simulink model "rate_control"  (R2024a)
settings: Solver=FixedStepAuto  StartTime=0  StopTime=TimeStop  FixedStep=TimeStep  RelTol=1e-3
values from neighbouring files (symbols this model uses):
  D = Y_bar(:,1:m)    [Auxi_OKID_JXL.m]    (also in limit_cycle_est.m = 0:0.01:1)
  Desire_att = [0;0;90]    [run_pwpf.m]
  filter_gain_z = 2    [run_pwpf.m]
  filter_time_constant_x = 0.1    [run_pwpf.m]
  filter_time_constant_y = 0.1    [run_pwpf.m]
  filter_time_constant_z = 0.5    [run_pwpf.m]
  I = [0.619 -0.008 0;-0.008 0.782 0;0 0 1.226]    [limit_cycle_est.m]    (also in moment_calculation.m; run_pwpf.m = 1*[0.619 -0.008 0;-0.008 0.782 0;0 0 1.226])
  initial_condition = [20;20;0]    [run_pwpf.m]
  Schimitt_Lower_bound_x = 0.15    [run_pwpf.m]
  Schimitt_Lower_bound_y = 0.15    [run_pwpf.m]
  Schimitt_Lower_bound_z = 0.15    [run_pwpf.m]
  Schimitt_Upper_bound_x = 0.5    [run_pwpf.m]
  Schimitt_Upper_bound_y = 0.5    [run_pwpf.m]
  Schimitt_Upper_bound_z = 3    [run_pwpf.m]
  Thruster_mom_x = 0.35*0.5    (= 0.175)    [run_pwpf.m]
  Thruster_mom_y = 0.35*0.5    (= 0.175)    [run_pwpf.m]
  Thruster_mom_z = 0.35*0.5*2    (= 0.35)    [run_pwpf.m]
undefined symbols (not defined in the file or in its folder): aMode
libraries: slpidlib x6, simulink_extras x4, shared6dofsys x1, sharedutil x1
settings Model: Creator=cnsl  LastModifiedBy=s3928
settings DebuggingCC: AlgebraicLoopMsg=none
settings RTWCC: GPUComputeCapability=3.5

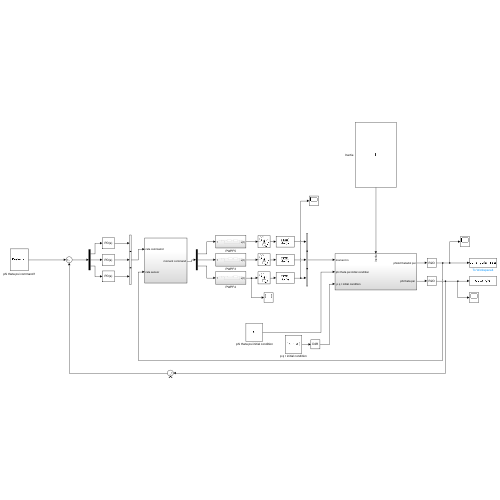
[thumbnail: Simulink's stored preview of the top-level diagram]
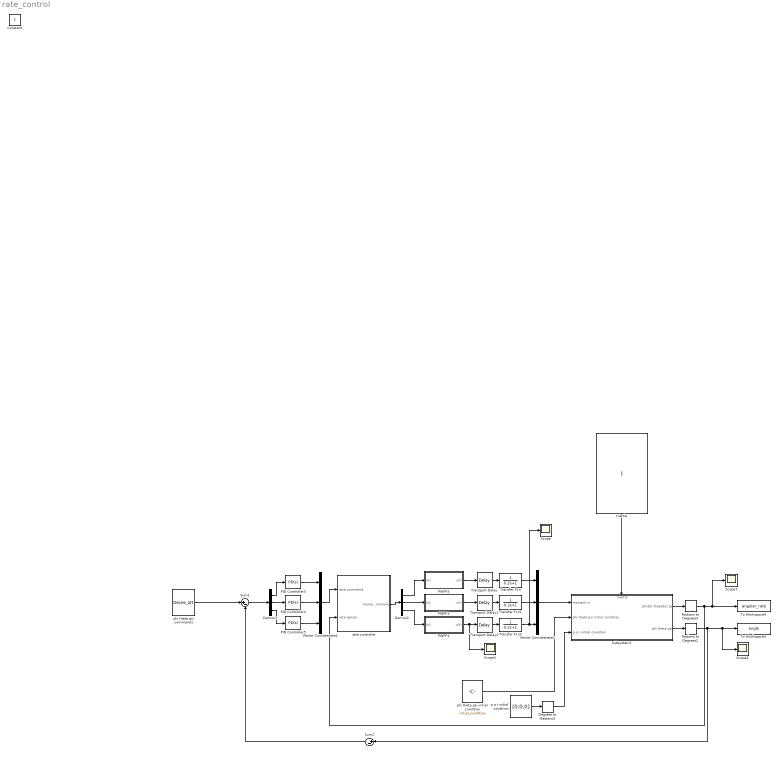
== system rate_control ==
  " phi theta psi initial condition" : Constant  Value=initial_condition
  Degrees to Radians3 : simulink_extras/Transformations/Degrees to Radians
  Demux1 : Demux  Outputs=3
  Demux2 : Demux  Outputs=3
  Inertie : Constant  Value=I
  PID Controller3 : slpidlib/PID Controller  Controller=PD  Form=Parallel  TimeDomain=Continuous-time  UseExternalTs=off  SampleTime=-1  IntegratorMethod=Forward Euler  FilterMethod=Forward Euler  ControllerParametersSource=internal  P=1  I=0.5  UseKiTs=off  D=2  UseExternalDerivativeSource=off  N=174.045132918495  UseFilter=on  TunerSelectOption=Transfer Function Based (PID Tuner App)  InitialConditionSource=internal  InitialConditionForIntegrator=0  InitialConditionForFilter=0  DifferentiatorICPrevScaledInput=0  ExternalReset=none  TrackingMode=off  Kt=1  LimitOutput=off  SatLimitsSource=internal  UpperSaturationLimit=inf  LowerSaturationLimit=-inf  LinearizeAsGain=on  AntiWindupMode=none  Kb=1  LimitIntegrator=off  UpperIntegratorSaturationLimit=inf  LowerIntegratorSaturationLimit=-inf  POutMin=[]  POutMax=[]  IOutMin=[]  IOutMax=[]  DOutMin=[]  DOutMax=[]  NOutMin=[]  NOutMax=[]  SumOutMin=[]  SumOutMax=[]  SaturationOutMin=[]  SaturationOutMax=[]  PParamMin=[]  PParamMax=[]  IParamMin=[]  IParamMax=[]  DParamMin=[]  DParamMax=[]  NParamMin=[]  NParamMax=[]  KbParamMin=[]  KbParamMax=[]  KtParamMin=[]  KtParamMax=[]  KbOutMin=[]  KbOutMax=[]  KtOutMin=[]  KtOutMax=[]  IntegratorOutMin=[]  IntegratorOutMax=[]  FilterOutMin=[]  FilterOutMax=[]  SumI1OutMin=[]  SumI1OutMax=[]  SumI2OutMin=[]  SumI2OutMax=[]  SumI3OutMin=[]  SumI3OutMax=[]  SumI4OutMin=[]  SumI4OutMax=[]  SumDOutMin=[]  SumDOutMax=[]  DifferentiatorOutMin=[]  DifferentiatorOutMax=[]  FilterDiffOutCoefMin=[]  FilterDiffOutCoefMax=[]  ReciprocalOutMin=[]  ReciprocalOutMax=[]  SumDenOutMin=[]  SumDenOutMax=[]  SumNumOutMin=[]  SumNumOutMax=[]  DivideOutMin=[]  DivideOutMax=[]  UdiffTsProdOutMin=[]  UdiffTsProdOutMax=[]  NTsProdOutMin=[]  NTsProdOutMax=[]  UintegralTsProdOutMin=[]  UintegralTsProdOutMax=[]  UngainTsProdOutMin=[]  UngainTsProdOutMax=[]  ClampingZeroOutDataTypeStr=Inherit: Inherit via back propagation  ClampingZeroOutMin=[]  ClampingZeroOutMax=[]  FilterDenConstantOutDataTypeStr=Inherit: Inherit via back propagation  FilterDenConstantOutMin=[]  FilterDenConstantOutMax=[]  PCopyOutDataTypeStr=Inherit: Inherit via back propagation  PCopyOutMin=[]  PCopyOutMax=[]  NCopyOutDataTypeStr=Inherit: Inherit via back propagation  NCopyOutMin=[]  NCopyOutMax=[]  IntegratorContinuousStateAttributes=''  IntegratorStateMustResolveToSignalObject=off  IntegratorRTWStateStorageClass=Auto  FilterContinuousStateAttributes=''  FilterStateMustResolveToSignalObject=off  FilterRTWStateStorageClass=Auto  ParallelPVariant=InternalParameters  IdealPVariant=Disabled  IVariant=Disabled  DVariant=InternalParameters  IntegratorVariant=Disabled  SatVariant=Disabled  AWVariant=Disabled  PCopyVariant=Disabled  TRVariant=Disabled  FdbkBlocksVariant=Forward  IdealPFdbkVariant=Disabled  SatFdbkVariant=Disabled  DerivativeFilterVariant=ContFilter  NVariant=InternalParameters  NCopyVariant=Disabled  FilterICVariant=InternalICsFilter  IntegratorICVariant=Disabled  ExternalResetVariant=Disabled  TRSumVariant=Passthrough  SumFdbkVariant=Disabled  SumVariant=Sum_PD  TsampFilterVariant=InternalTs  TsampNgainVariant=Passthrough  TsampIntegralVariant=Disabled_SignalSpec  ExternalSaturationOutDataTypeStr=Inherit: Same as second input  DerivativeSourceVariant=ErrorSignal
  PID Controller4 : slpidlib/PID Controller  Controller=PD  Form=Parallel  TimeDomain=Continuous-time  UseExternalTs=off  SampleTime=-1  IntegratorMethod=Forward Euler  FilterMethod=Forward Euler  ControllerParametersSource=internal  P=1  I=0.1  UseKiTs=off  D=2  UseExternalDerivativeSource=off  N=1000  UseFilter=on  TunerSelectOption=Transfer Function Based (PID Tuner App)  InitialConditionSource=internal  InitialConditionForIntegrator=0  InitialConditionForFilter=0  DifferentiatorICPrevScaledInput=0  ExternalReset=none  TrackingMode=off  Kt=1  LimitOutput=off  SatLimitsSource=internal  UpperSaturationLimit=inf  LowerSaturationLimit=-inf  LinearizeAsGain=on  AntiWindupMode=none  Kb=1  LimitIntegrator=off  UpperIntegratorSaturationLimit=inf  LowerIntegratorSaturationLimit=-inf  POutMin=[]  POutMax=[]  IOutMin=[]  IOutMax=[]  DOutMin=[]  DOutMax=[]  NOutMin=[]  NOutMax=[]  SumOutMin=[]  SumOutMax=[]  SaturationOutMin=[]  SaturationOutMax=[]  PParamMin=[]  PParamMax=[]  IParamMin=[]  IParamMax=[]  DParamMin=[]  DParamMax=[]  NParamMin=[]  NParamMax=[]  KbParamMin=[]  KbParamMax=[]  KtParamMin=[]  KtParamMax=[]  KbOutMin=[]  KbOutMax=[]  KtOutMin=[]  KtOutMax=[]  IntegratorOutMin=[]  IntegratorOutMax=[]  FilterOutMin=[]  FilterOutMax=[]  SumI1OutMin=[]  SumI1OutMax=[]  SumI2OutMin=[]  SumI2OutMax=[]  SumI3OutMin=[]  SumI3OutMax=[]  SumI4OutMin=[]  SumI4OutMax=[]  SumDOutMin=[]  SumDOutMax=[]  DifferentiatorOutMin=[]  DifferentiatorOutMax=[]  FilterDiffOutCoefMin=[]  FilterDiffOutCoefMax=[]  ReciprocalOutMin=[]  ReciprocalOutMax=[]  SumDenOutMin=[]  SumDenOutMax=[]  SumNumOutMin=[]  SumNumOutMax=[]  DivideOutMin=[]  DivideOutMax=[]  UdiffTsProdOutMin=[]  UdiffTsProdOutMax=[]  NTsProdOutMin=[]  NTsProdOutMax=[]  UintegralTsProdOutMin=[]  UintegralTsProdOutMax=[]  UngainTsProdOutMin=[]  UngainTsProdOutMax=[]  ClampingZeroOutDataTypeStr=Inherit: Inherit via back propagation  ClampingZeroOutMin=[]  ClampingZeroOutMax=[]  FilterDenConstantOutDataTypeStr=Inherit: Inherit via back propagation  FilterDenConstantOutMin=[]  FilterDenConstantOutMax=[]  PCopyOutDataTypeStr=Inherit: Inherit via back propagation  PCopyOutMin=[]  PCopyOutMax=[]  NCopyOutDataTypeStr=Inherit: Inherit via back propagation  NCopyOutMin=[]  NCopyOutMax=[]  IntegratorContinuousStateAttributes=''  IntegratorStateMustResolveToSignalObject=off  IntegratorRTWStateStorageClass=Auto  FilterContinuousStateAttributes=''  FilterStateMustResolveToSignalObject=off  FilterRTWStateStorageClass=Auto  ParallelPVariant=InternalParameters  IdealPVariant=Disabled  IVariant=Disabled  DVariant=InternalParameters  IntegratorVariant=Disabled  SatVariant=Disabled  AWVariant=Disabled  PCopyVariant=Disabled  TRVariant=Disabled  FdbkBlocksVariant=Forward  IdealPFdbkVariant=Disabled  SatFdbkVariant=Disabled  DerivativeFilterVariant=ContFilter  NVariant=InternalParameters  NCopyVariant=Disabled  FilterICVariant=InternalICsFilter  IntegratorICVariant=Disabled  ExternalResetVariant=Disabled  TRSumVariant=Passthrough  SumFdbkVariant=Disabled  SumVariant=Sum_PD  TsampFilterVariant=InternalTs  TsampNgainVariant=Passthrough  TsampIntegralVariant=Disabled_SignalSpec  ExternalSaturationOutDataTypeStr=Inherit: Same as second input  DerivativeSourceVariant=ErrorSignal
  PID Controller5 : slpidlib/PID Controller  Controller=PD  Form=Parallel  TimeDomain=Continuous-time  UseExternalTs=off  SampleTime=-1  IntegratorMethod=Forward Euler  FilterMethod=Forward Euler  ControllerParametersSource=internal  P=1  I=0.2  UseKiTs=off  D=2  UseExternalDerivativeSource=off  N=1142.8279760416  UseFilter=on  TunerSelectOption=Transfer Function Based (PID Tuner App)  InitialConditionSource=internal  InitialConditionForIntegrator=0  InitialConditionForFilter=0  DifferentiatorICPrevScaledInput=0  ExternalReset=none  TrackingMode=off  Kt=1  LimitOutput=off  SatLimitsSource=internal  UpperSaturationLimit=inf  LowerSaturationLimit=-inf  LinearizeAsGain=on  AntiWindupMode=none  Kb=1  LimitIntegrator=off  UpperIntegratorSaturationLimit=inf  LowerIntegratorSaturationLimit=-inf  POutMin=[]  POutMax=[]  IOutMin=[]  IOutMax=[]  DOutMin=[]  DOutMax=[]  NOutMin=[]  NOutMax=[]  SumOutMin=[]  SumOutMax=[]  SaturationOutMin=[]  SaturationOutMax=[]  PParamMin=[]  PParamMax=[]  IParamMin=[]  IParamMax=[]  DParamMin=[]  DParamMax=[]  NParamMin=[]  NParamMax=[]  KbParamMin=[]  KbParamMax=[]  KtParamMin=[]  KtParamMax=[]  KbOutMin=[]  KbOutMax=[]  KtOutMin=[]  KtOutMax=[]  IntegratorOutMin=[]  IntegratorOutMax=[]  FilterOutMin=[]  FilterOutMax=[]  SumI1OutMin=[]  SumI1OutMax=[]  SumI2OutMin=[]  SumI2OutMax=[]  SumI3OutMin=[]  SumI3OutMax=[]  SumI4OutMin=[]  SumI4OutMax=[]  SumDOutMin=[]  SumDOutMax=[]  DifferentiatorOutMin=[]  DifferentiatorOutMax=[]  FilterDiffOutCoefMin=[]  FilterDiffOutCoefMax=[]  ReciprocalOutMin=[]  ReciprocalOutMax=[]  SumDenOutMin=[]  SumDenOutMax=[]  SumNumOutMin=[]  SumNumOutMax=[]  DivideOutMin=[]  DivideOutMax=[]  UdiffTsProdOutMin=[]  UdiffTsProdOutMax=[]  NTsProdOutMin=[]  NTsProdOutMax=[]  UintegralTsProdOutMin=[]  UintegralTsProdOutMax=[]  UngainTsProdOutMin=[]  UngainTsProdOutMax=[]  ClampingZeroOutDataTypeStr=Inherit: Inherit via back propagation  ClampingZeroOutMin=[]  ClampingZeroOutMax=[]  FilterDenConstantOutDataTypeStr=Inherit: Inherit via back propagation  FilterDenConstantOutMin=[]  FilterDenConstantOutMax=[]  PCopyOutDataTypeStr=Inherit: Inherit via back propagation  PCopyOutMin=[]  PCopyOutMax=[]  NCopyOutDataTypeStr=Inherit: Inherit via back propagation  NCopyOutMin=[]  NCopyOutMax=[]  IntegratorContinuousStateAttributes=''  IntegratorStateMustResolveToSignalObject=off  IntegratorRTWStateStorageClass=Auto  FilterContinuousStateAttributes=''  FilterStateMustResolveToSignalObject=off  FilterRTWStateStorageClass=Auto  ParallelPVariant=InternalParameters  IdealPVariant=Disabled  IVariant=Disabled  DVariant=InternalParameters  IntegratorVariant=Disabled  SatVariant=Disabled  AWVariant=Disabled  PCopyVariant=Disabled  TRVariant=Disabled  FdbkBlocksVariant=Forward  IdealPFdbkVariant=Disabled  SatFdbkVariant=Disabled  DerivativeFilterVariant=ContFilter  NVariant=InternalParameters  NCopyVariant=Disabled  FilterICVariant=InternalICsFilter  IntegratorICVariant=Disabled  ExternalResetVariant=Disabled  TRSumVariant=Passthrough  SumFdbkVariant=Disabled  SumVariant=Sum_PD  TsampFilterVariant=InternalTs  TsampNgainVariant=Passthrough  TsampIntegralVariant=Disabled_SignalSpec  ExternalSaturationOutDataTypeStr=Inherit: Same as second input  DerivativeSourceVariant=ErrorSignal
  PWPF3 : Subsystem
  PWPF4 : Subsystem
  PWPF5 : Subsystem
  Radians to Degrees2 : simulink_extras/Transformations/Radians to Degrees
  Radians to Degrees3 : simulink_extras/Transformations/Radians to Degrees
  Scope{,1,3,7} (4 alike) : Scope
  Subsystem1 : Subsystem
      settings: PortSchema="{\"entries\":[{\"content\":{\"sides\":[{\"content\":{\"connectorIds\":[\"In1\",\"In2\",\"In3\"]},\"type\":\"ConnectorPlacement.EquallySpacedRectSide\",\"uuid\":\"69618b35-6270-4939-99e0-c93e8a624a88\"},{\"content\":{\"connectorIds\":[\"Out1\",\"Out2\"],\"side\":\"RIGHT\"},\"type\":\"ConnectorPlacement.EquallySpacedRectSide\",\"uuid\":\"dd38394a-61d4-4afa-a4aa-1d349921c55b\"},{\"content\":{\"connectorIds\":[\"In4\"],\"side\":\"TOP\"},\"type\":\"ConnectorPlacement.EquallySpacedRectSide\",\"uuid\":\"df8b2583-6705-491e-930f-9a3acb03c8ce\"}]},\"type\":\"ConnectorPlacement.EquallySpacedConnector\",\"uuid\":\"e8247de4-3909-4e19-8e9e-570170f34f7b\"}],\"packageUris\":[\"http://schema.mathworks.com/mf0/Connector/R2020b\"],\"version\":\"1.0\"}"
  Sum1 : Sum  Inputs=|+-
  Sum2 : Sum  Inputs=|+-
  To Workspace3 : ToWorkspace  VariableName=angle  SaveFormat=Timeseries  SampleTime=-1
  To Workspace4 : ToWorkspace  VariableName=angular_rate  SaveFormat=Timeseries  SampleTime=-1
  Transfer Fcn : TransferFcn  Denominator=[0.2 1]
  Transfer Fcn1 : TransferFcn  Denominator=[0.2 1]
  Transfer Fcn2 : TransferFcn  Denominator=[0.2 1]
  Transport Delay : TransportDelay  DelayTime=0.05
  Transport Delay1 : TransportDelay  DelayTime=0.05
  Transport Delay2 : TransportDelay  DelayTime=0.05
  Vector Concatenate1 : Concatenate  NumInputs=3
  Vector Concatenate2 : Concatenate  NumInputs=3
  p q r initial condition : Constant  Value=[0;0;0]
  phi theta psi command1 : Constant  Value=Desire_att
  rate controller : Subsystem
  Constant : Constant  IOType=siggen
  wires:
  Sum1/1 -> Demux1/1
  Demux1/2 -> PID Controller4/1
  Demux1/3 -> PID Controller5/1
  Subsystem1/1(phidot thetadot psi) -> Radians to Degrees3/1
  Demux1/1 -> PID Controller3/1
  phi theta psi command1/1 -> Sum1/1
  Subsystem1/2("phi theta psi ") -> Radians to Degrees2/1
  p q r initial condition/1 -> Degrees to Radians3/1
  Inertie/1 -> Subsystem1/4(inertia)
  Radians to Degrees3/1 -> rate controller/2(rate sensor), Scope7/1, To Workspace4/1
  " phi theta psi initial condition"/1 -> Subsystem1/2("phi theta psi initial condition ")
  Degrees to Radians3/1 -> Subsystem1/3(" p q r initial condition")
  Radians to Degrees2/1 -> Scope3/1, To Workspace3/1, Sum2/1
  PID Controller3/1 -> Vector Concatenate1/1
  PID Controller4/1 -> Vector Concatenate1/2
  PID Controller5/1 -> Vector Concatenate1/3
  Vector Concatenate1/1 -> rate controller/1(rate commamd)
  Demux2/1 -> PWPF5/1(In1)
  Demux2/3 -> PWPF4/1(In1)
  Demux2/2 -> PWPF3/1(In1)
  rate controller/1(moment command) -> Demux2/1
  Sum2/1 -> Sum1/2
  Vector Concatenate2/1 -> Subsystem1/1(moment in)
  Transport Delay/1 -> Transfer Fcn/1
  Transfer Fcn/1 -> Vector Concatenate2/1
  PWPF5/1(u(t)) -> Transport Delay/1
  Transport Delay1/1 -> Transfer Fcn1/1
  Transport Delay2/1 -> Transfer Fcn2/1
  Transfer Fcn1/1 -> Vector Concatenate2/2
  Transfer Fcn2/1 -> Scope/1, Vector Concatenate2/3
  PWPF3/1(u(t)) -> Transport Delay1/1
  PWPF4/1(u(t)) -> Scope1/1, Transport Delay2/1

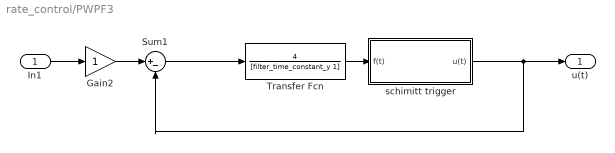
== system rate_control/PWPF3 ==
  In1 : Inport
  Gain2 : Gain
  Sum1 : Sum  Inputs=|+-
  Transfer Fcn : TransferFcn  Numerator=[4]  Denominator=[filter_time_constant_y 1]
  schimitt trigger : Subsystem
  u(t) : Outport
  wires:
  In1/1 -> Gain2/1
  Gain2/1 -> Sum1/1
  schimitt trigger/1(u(t)) -> u(t)/1, Sum1/2
  Sum1/1 -> Transfer Fcn/1
  Transfer Fcn/1 -> schimitt trigger/1(f(t))

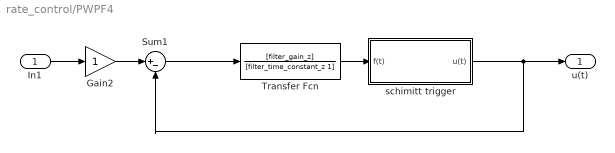
== system rate_control/PWPF4 ==
  In1 : Inport
  Gain2 : Gain
  Sum1 : Sum  Inputs=|+-
  Transfer Fcn : TransferFcn  Numerator=[filter_gain_z]  Denominator=[filter_time_constant_z 1]
  schimitt trigger : Subsystem
  u(t) : Outport
  wires:
  Transfer Fcn/1 -> schimitt trigger/1(f(t))
  Sum1/1 -> Transfer Fcn/1
  schimitt trigger/1(u(t)) -> Sum1/2, u(t)/1
  Gain2/1 -> Sum1/1
  In1/1 -> Gain2/1

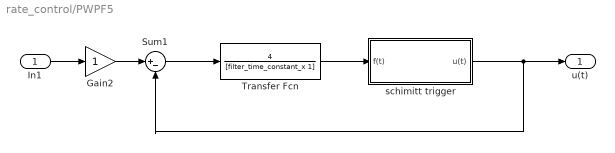
== system rate_control/PWPF5 ==
  In1 : Inport
  Gain2 : Gain
  Sum1 : Sum  Inputs=|+-
  Transfer Fcn : TransferFcn  Numerator=[4]  Denominator=[filter_time_constant_x 1]
  schimitt trigger : Subsystem
  u(t) : Outport
  wires:
  Transfer Fcn/1 -> schimitt trigger/1(f(t))
  Sum1/1 -> Transfer Fcn/1
  schimitt trigger/1(u(t)) -> Sum1/2, u(t)/1
  Gain2/1 -> Sum1/1
  In1/1 -> Gain2/1

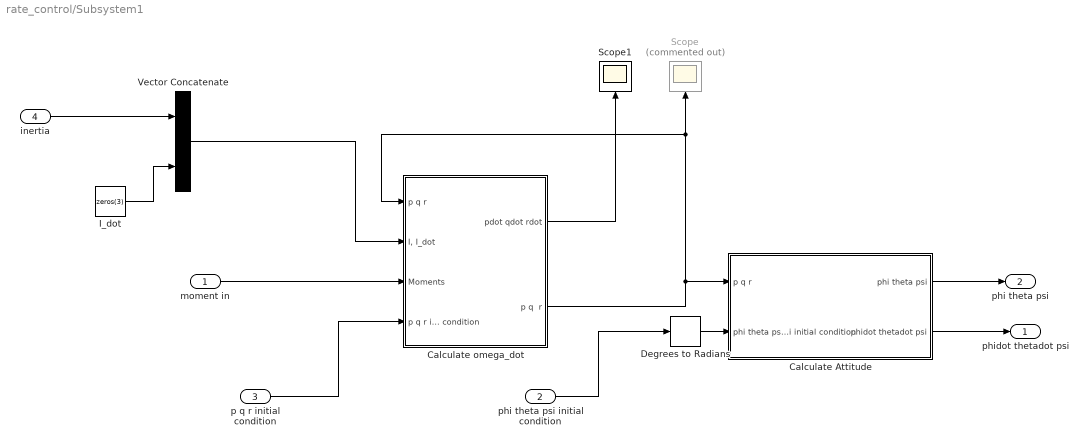
== system rate_control/Subsystem1 ==
  moment in : Inport
  "phi theta psi initial condition " : Inport  Port=2
  " p q r initial condition" : Inport  Port=3
  inertia : Inport  Port=4
  "Calculate Attitude " : Subsystem
  Calculate omega_dot : Subsystem  AncestorBlock=shared6dofsys/Calculate omega_dot  mask{aMode=aMode}
      mask init:
      | if aerosharedtest(gcb)
      |     aerosharedicon('shared');
      | else
      |     sharedautoicon('shared');
      | end
      settings: LibrarySourceBlock=shared6dofsys/Calculate omega_dot
  Degrees to Radians : simulink_extras/Transformations/Degrees to Radians
  I_dot : Constant  Value=zeros(3)
  Scope : Scope  Commented=on
  Scope1 : Scope
  Vector Concatenate : Concatenate  Mode=Multidimensional array
  phidot thetadot psi : Outport
  "phi theta psi " : Outport  Port=2
  wires:
  Vector Concatenate/1 -> Calculate omega_dot/2("I, I_dot")
  inertia/1 -> Vector Concatenate/1
  Calculate omega_dot/2(p q  r) -> Scope/1, Calculate omega_dot/1(p q r), "Calculate Attitude "/1(p q r)
  I_dot/1 -> Vector Concatenate/2
  " p q r initial condition"/1 -> Calculate omega_dot/4(p q r initial condition)
  "Calculate Attitude "/1("phi theta psi ") -> "phi theta psi "/1
  Degrees to Radians/1 -> "Calculate Attitude "/2("phi theta psi initial condition ")
  "phi theta psi initial condition "/1 -> Degrees to Radians/1
  "Calculate Attitude "/2(phidot thetadot psi) -> phidot thetadot psi/1
  Calculate omega_dot/1(pdot qdot rdot) -> Scope1/1
  moment in/1 -> Calculate omega_dot/3(Moments)

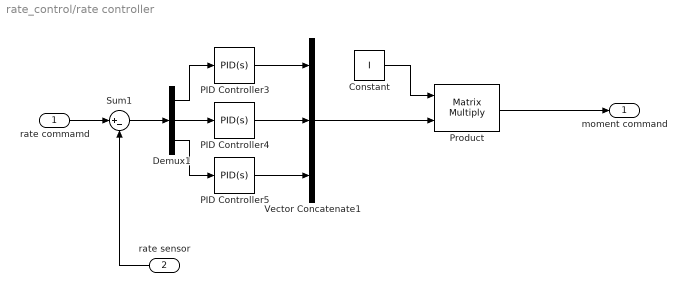
== system rate_control/rate controller ==
  rate commamd : Inport
  rate sensor : Inport  Port=2
  Constant : Constant  Value=I
  Demux1 : Demux  Outputs=3
  PID Controller3 : slpidlib/PID Controller  Controller=PID  Form=Parallel  TimeDomain=Continuous-time  UseExternalTs=off  SampleTime=-1  IntegratorMethod=Forward Euler  FilterMethod=Forward Euler  ControllerParametersSource=internal  P=2  I=0.25  UseKiTs=off  D=1  UseExternalDerivativeSource=off  N=100  UseFilter=on  TunerSelectOption=Transfer Function Based (PID Tuner App)  InitialConditionSource=internal  InitialConditionForIntegrator=0  InitialConditionForFilter=0  DifferentiatorICPrevScaledInput=0  ExternalReset=none  TrackingMode=off  Kt=1  LimitOutput=off  SatLimitsSource=internal  UpperSaturationLimit=inf  LowerSaturationLimit=-inf  LinearizeAsGain=on  AntiWindupMode=none  Kb=1  LimitIntegrator=off  UpperIntegratorSaturationLimit=inf  LowerIntegratorSaturationLimit=-inf  POutMin=[]  POutMax=[]  IOutMin=[]  IOutMax=[]  DOutMin=[]  DOutMax=[]  NOutMin=[]  NOutMax=[]  SumOutMin=[]  SumOutMax=[]  SaturationOutMin=[]  SaturationOutMax=[]  PParamMin=[]  PParamMax=[]  IParamMin=[]  IParamMax=[]  DParamMin=[]  DParamMax=[]  NParamMin=[]  NParamMax=[]  KbParamMin=[]  KbParamMax=[]  KtParamMin=[]  KtParamMax=[]  KbOutMin=[]  KbOutMax=[]  KtOutMin=[]  KtOutMax=[]  IntegratorOutMin=[]  IntegratorOutMax=[]  FilterOutMin=[]  FilterOutMax=[]  SumI1OutMin=[]  SumI1OutMax=[]  SumI2OutMin=[]  SumI2OutMax=[]  SumI3OutMin=[]  SumI3OutMax=[]  SumI4OutMin=[]  SumI4OutMax=[]  SumDOutMin=[]  SumDOutMax=[]  DifferentiatorOutMin=[]  DifferentiatorOutMax=[]  FilterDiffOutCoefMin=[]  FilterDiffOutCoefMax=[]  ReciprocalOutMin=[]  ReciprocalOutMax=[]  SumDenOutMin=[]  SumDenOutMax=[]  SumNumOutMin=[]  SumNumOutMax=[]  DivideOutMin=[]  DivideOutMax=[]  UdiffTsProdOutMin=[]  UdiffTsProdOutMax=[]  NTsProdOutMin=[]  NTsProdOutMax=[]  UintegralTsProdOutMin=[]  UintegralTsProdOutMax=[]  UngainTsProdOutMin=[]  UngainTsProdOutMax=[]  ClampingZeroOutDataTypeStr=Inherit: Inherit via back propagation  ClampingZeroOutMin=[]  ClampingZeroOutMax=[]  FilterDenConstantOutDataTypeStr=Inherit: Inherit via back propagation  FilterDenConstantOutMin=[]  FilterDenConstantOutMax=[]  PCopyOutDataTypeStr=Inherit: Inherit via back propagation  PCopyOutMin=[]  PCopyOutMax=[]  NCopyOutDataTypeStr=Inherit: Inherit via back propagation  NCopyOutMin=[]  NCopyOutMax=[]  IntegratorContinuousStateAttributes=''  IntegratorStateMustResolveToSignalObject=off  IntegratorRTWStateStorageClass=Auto  FilterContinuousStateAttributes=''  FilterStateMustResolveToSignalObject=off  FilterRTWStateStorageClass=Auto  ParallelPVariant=InternalParameters  IdealPVariant=Disabled  IVariant=InternalParameters  DVariant=InternalParameters  IntegratorVariant=Continuous  SatVariant=Disabled  AWVariant=Passthrough  PCopyVariant=Disabled  TRVariant=Disabled  FdbkBlocksVariant=Forward  IdealPFdbkVariant=Disabled  SatFdbkVariant=Disabled  DerivativeFilterVariant=ContFilter  NVariant=InternalParameters  NCopyVariant=Disabled  FilterICVariant=InternalICsFilter  IntegratorICVariant=InternalICs  ExternalResetVariant=Disabled  TRSumVariant=Passthrough  SumFdbkVariant=Disabled  SumVariant=Sum_PID  TsampFilterVariant=InternalTs  TsampNgainVariant=Passthrough  TsampIntegralVariant=Disabled_SignalSpec  ExternalSaturationOutDataTypeStr=Inherit: Same as second input  DerivativeSourceVariant=ErrorSignal
  PID Controller4 : slpidlib/PID Controller  Controller=PID  Form=Parallel  TimeDomain=Continuous-time  UseExternalTs=off  SampleTime=-1  IntegratorMethod=Forward Euler  FilterMethod=Forward Euler  ControllerParametersSource=internal  P=2  I=0.25  UseKiTs=off  D=1  UseExternalDerivativeSource=off  N=100  UseFilter=on  TunerSelectOption=Transfer Function Based (PID Tuner App)  InitialConditionSource=internal  InitialConditionForIntegrator=0  InitialConditionForFilter=0  DifferentiatorICPrevScaledInput=0  ExternalReset=none  TrackingMode=off  Kt=1  LimitOutput=off  SatLimitsSource=internal  UpperSaturationLimit=inf  LowerSaturationLimit=-inf  LinearizeAsGain=on  AntiWindupMode=none  Kb=1  LimitIntegrator=off  UpperIntegratorSaturationLimit=inf  LowerIntegratorSaturationLimit=-inf  POutMin=[]  POutMax=[]  IOutMin=[]  IOutMax=[]  DOutMin=[]  DOutMax=[]  NOutMin=[]  NOutMax=[]  SumOutMin=[]  SumOutMax=[]  SaturationOutMin=[]  SaturationOutMax=[]  PParamMin=[]  PParamMax=[]  IParamMin=[]  IParamMax=[]  DParamMin=[]  DParamMax=[]  NParamMin=[]  NParamMax=[]  KbParamMin=[]  KbParamMax=[]  KtParamMin=[]  KtParamMax=[]  KbOutMin=[]  KbOutMax=[]  KtOutMin=[]  KtOutMax=[]  IntegratorOutMin=[]  IntegratorOutMax=[]  FilterOutMin=[]  FilterOutMax=[]  SumI1OutMin=[]  SumI1OutMax=[]  SumI2OutMin=[]  SumI2OutMax=[]  SumI3OutMin=[]  SumI3OutMax=[]  SumI4OutMin=[]  SumI4OutMax=[]  SumDOutMin=[]  SumDOutMax=[]  DifferentiatorOutMin=[]  DifferentiatorOutMax=[]  FilterDiffOutCoefMin=[]  FilterDiffOutCoefMax=[]  ReciprocalOutMin=[]  ReciprocalOutMax=[]  SumDenOutMin=[]  SumDenOutMax=[]  SumNumOutMin=[]  SumNumOutMax=[]  DivideOutMin=[]  DivideOutMax=[]  UdiffTsProdOutMin=[]  UdiffTsProdOutMax=[]  NTsProdOutMin=[]  NTsProdOutMax=[]  UintegralTsProdOutMin=[]  UintegralTsProdOutMax=[]  UngainTsProdOutMin=[]  UngainTsProdOutMax=[]  ClampingZeroOutDataTypeStr=Inherit: Inherit via back propagation  ClampingZeroOutMin=[]  ClampingZeroOutMax=[]  FilterDenConstantOutDataTypeStr=Inherit: Inherit via back propagation  FilterDenConstantOutMin=[]  FilterDenConstantOutMax=[]  PCopyOutDataTypeStr=Inherit: Inherit via back propagation  PCopyOutMin=[]  PCopyOutMax=[]  NCopyOutDataTypeStr=Inherit: Inherit via back propagation  NCopyOutMin=[]  NCopyOutMax=[]  IntegratorContinuousStateAttributes=''  IntegratorStateMustResolveToSignalObject=off  IntegratorRTWStateStorageClass=Auto  FilterContinuousStateAttributes=''  FilterStateMustResolveToSignalObject=off  FilterRTWStateStorageClass=Auto  ParallelPVariant=InternalParameters  IdealPVariant=Disabled  IVariant=InternalParameters  DVariant=InternalParameters  IntegratorVariant=Continuous  SatVariant=Disabled  AWVariant=Passthrough  PCopyVariant=Disabled  TRVariant=Disabled  FdbkBlocksVariant=Forward  IdealPFdbkVariant=Disabled  SatFdbkVariant=Disabled  DerivativeFilterVariant=ContFilter  NVariant=InternalParameters  NCopyVariant=Disabled  FilterICVariant=InternalICsFilter  IntegratorICVariant=InternalICs  ExternalResetVariant=Disabled  TRSumVariant=Passthrough  SumFdbkVariant=Disabled  SumVariant=Sum_PID  TsampFilterVariant=InternalTs  TsampNgainVariant=Passthrough  TsampIntegralVariant=Disabled_SignalSpec  ExternalSaturationOutDataTypeStr=Inherit: Same as second input  DerivativeSourceVariant=ErrorSignal
  PID Controller5 : slpidlib/PID Controller  Controller=PID  Form=Parallel  TimeDomain=Continuous-time  UseExternalTs=off  SampleTime=-1  IntegratorMethod=Forward Euler  FilterMethod=Forward Euler  ControllerParametersSource=internal  P=2  I=0.25  UseKiTs=off  D=1  UseExternalDerivativeSource=off  N=100  UseFilter=on  TunerSelectOption=Transfer Function Based (PID Tuner App)  InitialConditionSource=internal  InitialConditionForIntegrator=0  InitialConditionForFilter=0  DifferentiatorICPrevScaledInput=0  ExternalReset=none  TrackingMode=off  Kt=1  LimitOutput=off  SatLimitsSource=internal  UpperSaturationLimit=inf  LowerSaturationLimit=-inf  LinearizeAsGain=on  AntiWindupMode=none  Kb=1  LimitIntegrator=off  UpperIntegratorSaturationLimit=inf  LowerIntegratorSaturationLimit=-inf  POutMin=[]  POutMax=[]  IOutMin=[]  IOutMax=[]  DOutMin=[]  DOutMax=[]  NOutMin=[]  NOutMax=[]  SumOutMin=[]  SumOutMax=[]  SaturationOutMin=[]  SaturationOutMax=[]  PParamMin=[]  PParamMax=[]  IParamMin=[]  IParamMax=[]  DParamMin=[]  DParamMax=[]  NParamMin=[]  NParamMax=[]  KbParamMin=[]  KbParamMax=[]  KtParamMin=[]  KtParamMax=[]  KbOutMin=[]  KbOutMax=[]  KtOutMin=[]  KtOutMax=[]  IntegratorOutMin=[]  IntegratorOutMax=[]  FilterOutMin=[]  FilterOutMax=[]  SumI1OutMin=[]  SumI1OutMax=[]  SumI2OutMin=[]  SumI2OutMax=[]  SumI3OutMin=[]  SumI3OutMax=[]  SumI4OutMin=[]  SumI4OutMax=[]  SumDOutMin=[]  SumDOutMax=[]  DifferentiatorOutMin=[]  DifferentiatorOutMax=[]  FilterDiffOutCoefMin=[]  FilterDiffOutCoefMax=[]  ReciprocalOutMin=[]  ReciprocalOutMax=[]  SumDenOutMin=[]  SumDenOutMax=[]  SumNumOutMin=[]  SumNumOutMax=[]  DivideOutMin=[]  DivideOutMax=[]  UdiffTsProdOutMin=[]  UdiffTsProdOutMax=[]  NTsProdOutMin=[]  NTsProdOutMax=[]  UintegralTsProdOutMin=[]  UintegralTsProdOutMax=[]  UngainTsProdOutMin=[]  UngainTsProdOutMax=[]  ClampingZeroOutDataTypeStr=Inherit: Inherit via back propagation  ClampingZeroOutMin=[]  ClampingZeroOutMax=[]  FilterDenConstantOutDataTypeStr=Inherit: Inherit via back propagation  FilterDenConstantOutMin=[]  FilterDenConstantOutMax=[]  PCopyOutDataTypeStr=Inherit: Inherit via back propagation  PCopyOutMin=[]  PCopyOutMax=[]  NCopyOutDataTypeStr=Inherit: Inherit via back propagation  NCopyOutMin=[]  NCopyOutMax=[]  IntegratorContinuousStateAttributes=''  IntegratorStateMustResolveToSignalObject=off  IntegratorRTWStateStorageClass=Auto  FilterContinuousStateAttributes=''  FilterStateMustResolveToSignalObject=off  FilterRTWStateStorageClass=Auto  ParallelPVariant=InternalParameters  IdealPVariant=Disabled  IVariant=InternalParameters  DVariant=InternalParameters  IntegratorVariant=Continuous  SatVariant=Disabled  AWVariant=Passthrough  PCopyVariant=Disabled  TRVariant=Disabled  FdbkBlocksVariant=Forward  IdealPFdbkVariant=Disabled  SatFdbkVariant=Disabled  DerivativeFilterVariant=ContFilter  NVariant=InternalParameters  NCopyVariant=Disabled  FilterICVariant=InternalICsFilter  IntegratorICVariant=InternalICs  ExternalResetVariant=Disabled  TRSumVariant=Passthrough  SumFdbkVariant=Disabled  SumVariant=Sum_PID  TsampFilterVariant=InternalTs  TsampNgainVariant=Passthrough  TsampIntegralVariant=Disabled_SignalSpec  ExternalSaturationOutDataTypeStr=Inherit: Same as second input  DerivativeSourceVariant=ErrorSignal
  Product : Product  Multiplication=Matrix(*)
  Sum1 : Sum  Inputs=|+-
  Vector Concatenate1 : Concatenate  NumInputs=3
  moment command : Outport
  wires:
  Demux1/3 -> PID Controller5/1
  Demux1/2 -> PID Controller4/1
  Demux1/1 -> PID Controller3/1
  PID Controller3/1 -> Vector Concatenate1/1
  PID Controller4/1 -> Vector Concatenate1/2
  PID Controller5/1 -> Vector Concatenate1/3
  Vector Concatenate1/1 -> Product/2
  Constant/1 -> Product/1
  Product/1 -> moment command/1
  Sum1/1 -> Demux1/1
  rate commamd/1 -> Sum1/1
  rate sensor/1 -> Sum1/2

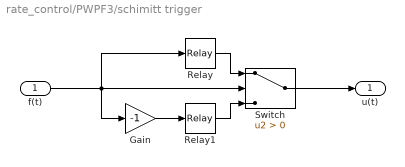
== system rate_control/PWPF3/schimitt trigger ==
  f(t) : Inport
  Gain : Gain  Gain=-1
  Relay : Relay  OnSwitchValue=Schimitt_Upper_bound_y  OffSwitchValue=Schimitt_Lower_bound_y  OnOutputValue=Thruster_mom_y
  Relay1 : Relay  OnSwitchValue=Schimitt_Upper_bound_y  OffSwitchValue=Schimitt_Lower_bound_y  OnOutputValue=-Thruster_mom_y
  Switch : Switch  Criteria=u2 > Threshold  SaturateOnIntegerOverflow=off  InputSameDT=off
  u(t) : Outport
  wires:
  Switch/1 -> u(t)/1
  Relay/1 -> Switch/1
  Gain/1 -> Relay1/1
  Relay1/1 -> Switch/3
  f(t)/1 -> Switch/2, Gain/1, Relay/1

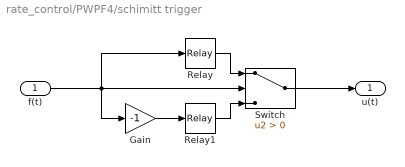
== system rate_control/PWPF4/schimitt trigger ==
  f(t) : Inport
  Gain : Gain  Gain=-1
  Relay : Relay  OnSwitchValue=Schimitt_Upper_bound_z  OffSwitchValue=Schimitt_Lower_bound_z  OnOutputValue=Thruster_mom_z
  Relay1 : Relay  OnSwitchValue=Schimitt_Upper_bound_z  OffSwitchValue=Schimitt_Lower_bound_z  OnOutputValue=-Thruster_mom_z
  Switch : Switch  Criteria=u2 > Threshold  SaturateOnIntegerOverflow=off  InputSameDT=off
  u(t) : Outport
  wires:
  f(t)/1 -> Relay/1, Gain/1, Switch/2
  Relay1/1 -> Switch/3
  Gain/1 -> Relay1/1
  Relay/1 -> Switch/1
  Switch/1 -> u(t)/1

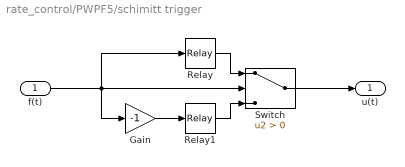
== system rate_control/PWPF5/schimitt trigger ==
  f(t) : Inport
  Gain : Gain  Gain=-1
  Relay : Relay  OnSwitchValue=Schimitt_Upper_bound_x  OffSwitchValue=Schimitt_Lower_bound_x  OnOutputValue=Thruster_mom_x
  Relay1 : Relay  OnSwitchValue=Schimitt_Upper_bound_x  OffSwitchValue=Schimitt_Lower_bound_x  OnOutputValue=-Thruster_mom_x
  Switch : Switch  Criteria=u2 > Threshold  SaturateOnIntegerOverflow=off  InputSameDT=off
  u(t) : Outport
  wires:
  f(t)/1 -> Relay/1, Gain/1, Switch/2
  Relay1/1 -> Switch/3
  Gain/1 -> Relay1/1
  Relay/1 -> Switch/1
  Switch/1 -> u(t)/1

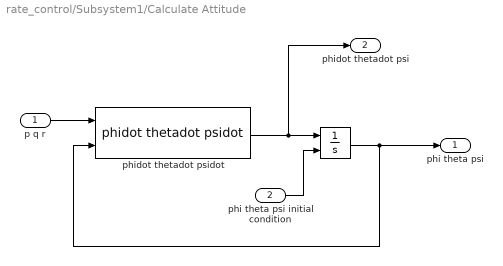
== system rate_control/Subsystem1/Calculate Attitude  ==
  p q r : Inport
  "phi theta psi initial condition " : Inport  Port=2
  " " : Integrator  InitialConditionSource=external
  phidot thetadot psidot : shared6dofsys/DCM & Euler Angles (Euler)/phidot thetadot psidot  SystemSampleTime=-1  VariantActivationTime=update diagram  AllowFlexibleInterface=on  Latency=0  AutoFrameSizeCalculation=off
  "phi theta psi " : Outport
  phidot thetadot psi : Outport  Port=2
  wires:
  "phi theta psi initial condition "/1 -> " "/2
  " "/1 -> phidot thetadot psidot/2, "phi theta psi "/1
  phidot thetadot psidot/1 -> phidot thetadot psi/1, " "/1
  p q r/1 -> phidot thetadot psidot/1

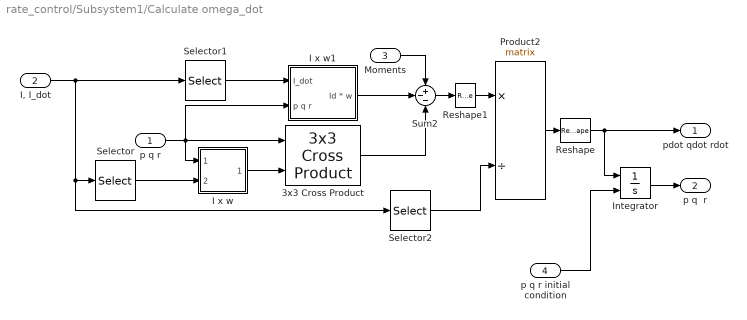
== system rate_control/Subsystem1/Calculate omega_dot ==
  p q r : Inport  OutDataTypeStr=double
  "I, I_dot" : Inport  Port=2  OutDataTypeStr=double
  Moments : Inport  Port=3  OutDataTypeStr=double
  p q r initial condition : Inport  Port=4
  3x3 Cross Product : sharedutil/3x3 Cross Product  aMode=aMode
  I x w : Subsystem
  I x w1 : Subsystem
  Integrator : Integrator  InitialConditionSource=external
  Product2 : Product  Inputs=*/  Multiplication=Matrix(*)  SaturateOnIntegerOverflow=on  OutDataTypeStr=Inherit: Same as first input
  Reshape : Reshape
  Reshape1 : Reshape  OutputDimensionality=Row vector (2-D)
  Selector : Selector  NumberOfDimensions=2  InputPortWidth=2  IndexOptions=Index vector (dialog),Select all  Indices=1:3,-1  OutputSizes=1
  Selector1 : Selector  NumberOfDimensions=2  InputPortWidth=2  IndexOptions=Index vector (dialog),Select all  Indices=4:6,-1  OutputSizes=1
  Selector2 : Selector  NumberOfDimensions=2  InputPortWidth=2  IndexOptions=Index vector (dialog),Select all  Indices=1:3,-1  OutputSizes=1
  Sum2 : Sum  Inputs=+--  SaturateOnIntegerOverflow=on
  pdot qdot rdot : Outport  OutDataTypeStr=double  VectorParamsAs1DForOutWhenUnconnected=off
  p q  r : Outport  Port=2
  wires:
  p q r initial condition/1 -> Integrator/2
  Integrator/1 -> p q  r/1
  Reshape/1 -> pdot qdot rdot/1, Integrator/1
  Selector/1 -> I x w/2(Inertia)
  Selector2/1 -> Product2/2
  "I, I_dot"/1 -> Selector/1, Selector2/1, Selector1/1
  p q r/1 -> 3x3 Cross Product/1, I x w1/2(p q r), I x w/1(p q r)
  Product2/1 -> Reshape/1
  Sum2/1 -> Reshape1/1
  Moments/1 -> Sum2/1
  I x w1/1(Id * w) -> Sum2/2
  Selector1/1 -> I x w1/1(I_dot)
  I x w/1(I * w) -> 3x3 Cross Product/2
  Reshape1/1 -> Product2/1
  3x3 Cross Product/1 -> Sum2/3

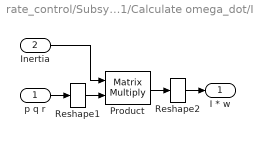
== system rate_control/Subsystem1/Calculate omega_dot/I x w ==
  p q r : Inport
  Inertia : Inport  Port=2
  Product : Product  Multiplication=Matrix(*)  InputSameDT=on  SaturateOnIntegerOverflow=on  OutDataTypeStr=Inherit: Same as first input
  Reshape1 : Reshape  OutputDimensionality=Column vector (2-D)
  Reshape2 : Reshape
  I * w : Outport  VectorParamsAs1DForOutWhenUnconnected=off
  wires:
  Product/1 -> Reshape2/1
  Inertia/1 -> Product/1
  p q r/1 -> Reshape1/1
  Reshape1/1 -> Product/2
  Reshape2/1 -> I * w/1

== system rate_control/Subsystem1/Calculate omega_dot/I x w1 ==
  I_dot : Inport
  p q r : Inport  Port=2
  Product : Product  Multiplication=Matrix(*)  InputSameDT=on  SaturateOnIntegerOverflow=on  OutDataTypeStr=Inherit: Same as first input
  Reshape1 : Reshape  OutputDimensionality=Column vector (2-D)
  Reshape2 : Reshape
  Id * w : Outport  VectorParamsAs1DForOutWhenUnconnected=off
  wires:
  p q r/1 -> Reshape1/1
  I_dot/1 -> Product/1
  Product/1 -> Reshape2/1
  Reshape1/1 -> Product/2
  Reshape2/1 -> Id * w/1
